simulink model "gm_CSC"  (R2016a)
settings: Solver=FixedStepDiscrete  SolverMode=SingleTasking  StartTime=0.0  StopTime=image_sample_time  RelTol=1e-3
PreLoadFcn:
  | R=105;
  | C=160;
  | Ts = 1/10;
  | image_sample_time = R*C/10;
undefined symbols (not defined in the file or in its folder): gray
libraries: hdlsllib x11, dspsigattribs x2, simulink x2, visionsources x1
Description:
  | Sobel Edge Detection Using the MATLAB(R) Function Block
  | This example shows how to use HDL Coder(TM) to check,
  | generate, and verify HDL code for a Sobel Edge Detection
  | block built using the MATLAB Function block.
settings Model: FPTRunName=Active  Creator=abehbood  LastModifiedBy=KAU-Sprinter
settings DataIOCC: LimitDataPoints=on  SaveFormat=Array  SignalLogging=off
settings OptimizationCC: BlockReduction=off  ConditionallyExecuteInputs=off  DefaultParameterBehavior=Inlined  ExpressionDepthLimit=2147483647  InitFltsAndDblsToZero=on  EfficientMapNaN2IntZero=off
settings DebuggingCC: AlgebraicLoopMsg=error  SaveWithParameterizedLinksMsg=none  UnderspecifiedInitializationDetection=Classic  MergeDetectMultiDrivingBlocksExec=none  SignalResolutionControl=TryResolveAllWithWarning  InheritedTsInSrcMsg=none  MultiTaskDSMMsg=warning  MultiTaskCondExecSysMsg=none  SingleTaskRateTransMsg=error  IntegerOverflowMsg=none  ParameterPrecisionLossMsg=none  FcnCallInpInsideContextMsg=UseLocalSettings  StateNameClashWarn=warning  StrictBusMsg=ErrorOnBusTreatedAsVector  IntegerSaturationMsg=none
settings HardwareCC: ProdBitPerPointer=32  ProdLargestAtomicFloat=None  ProdIntDivRoundTo=Undefined  ProdEndianess=Unspecified  ProdWordSize=32  ProdHWDeviceType=ASIC/FPGA  TargetHWDeviceType=32-bit Generic  ProdEqTarget=off
settings ModelReferenceCC: PropagateSignalLabelsOutOfModel=off
settings GRTTargetCC: TargetFcnLib=ansi_tfl_tmw.mat  CombineOutputUpdateFcns=off  GRTInterface=on
settings ConfigComp: CovModelRefEnable=Off

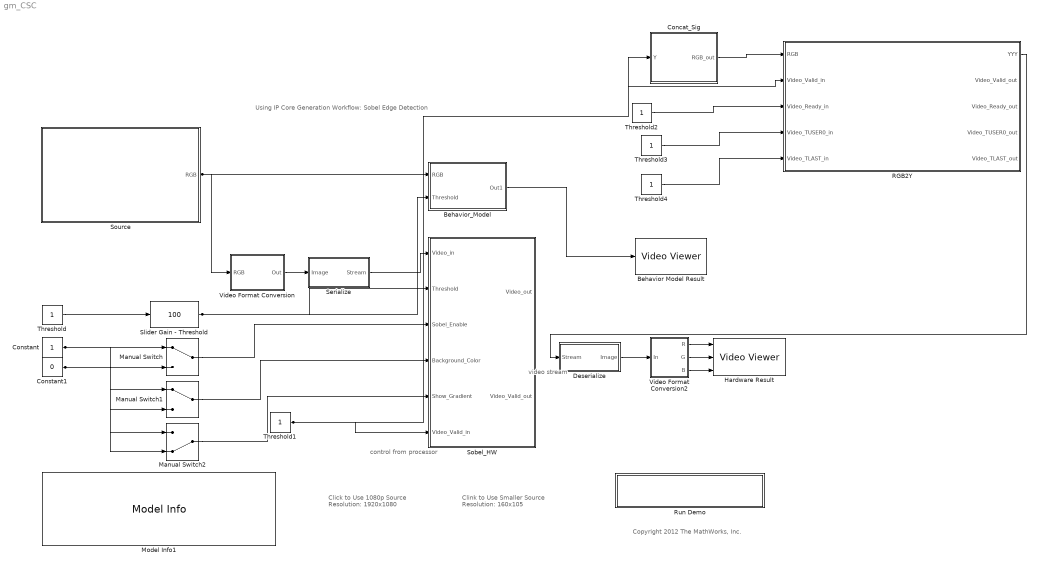
== system gm_CSC ==
  note: control from
      | processor
  note: video
      | stream
  note: Using IP Core Generation Workflow: Sobel Edge Detection
  note: Copyright 2012 The MathWorks, Inc.
  note: Clink to Use Smaller Source
      |
      | Resolution: 160x105
  note: Click to Use 1080p Source
      |
      | Resolution: 1920x1080
  Behavior Model Result : VideoViewer  colormapValue=gray(256)  FigPos=[941 500.4 363.2 159.2]
  Behavior_Model : Subsystem
  Concat_Sig : MATLAB Function  TreatAsAtomicUnit=on
  Constant : Constant  OutDataTypeStr=boolean  SampleTime=Ts
  Constant1 : Constant  Value=0  OutDataTypeStr=boolean  SampleTime=Ts
  Deserialize : Subsystem
  Hardware Result : VideoViewer  imagePorts=separate color signals  colormapValue=gray(256)  FigPos=[1151.4 744.4 360.8 160]
  Manual Switch : ManualSwitch
  Manual Switch1 : ManualSwitch
  Manual Switch2 : ManualSwitch  CurrentSetting=0
  Model Info1 : simulink/Model-Wide Utilities/Model Info  Frame=on  DisplayStringWithTags=|  HorizontalTextAlignment=Left  LeftAlignmentValue=0.02  SourceBlockDiagram=gm_CSC  TagMaxNumber=20
      | This example shows how to use HDL Coder to
      | generate a custom IP core which perform Sobel
      | edge detection processing on streaming video.
      | 
      | In MATLAB, type the following:
      |   hdladvisor('hdlcoder_sobel_video/Sobel_HW')
  RGB2Y : Subsystem  TreatAsAtomicUnit=on
  Run Demo : Subsystem
      settings: OpenFcn=hdladvisor([bdroot, '/Sobel_HW'])
      mask Display: disp('Launch HDL Workflow Advisor')
  Serialize : Subsystem
  Slider Gain - Threshold : simulink/Math Operations/Slider Gain  low=0  gain=100  high=255
  Sobel_HW : Subsystem  TreatAsAtomicUnit=on
  Source : Subsystem
      mask Display: image(imread('hdlcoder_sobel_160_105.jpg'))
  Threshold : Constant  OutDataTypeStr=uint8  SampleTime=Ts
  Threshold{1..4} (4 alike) : Constant  OutDataTypeStr=boolean  SampleTime=Ts
  Video Format Conversion : Subsystem
  Video Format Conversion2 : Subsystem
  wires:
  Threshold4/1 -> RGB2Y/5(Video_TLAST_in)
  Threshold3/1 -> RGB2Y/4(Video_TUSER0_in)
  Threshold2/1 -> RGB2Y/3(Video_Ready_in)
  Concat_Sig/1(RGB_out) -> RGB2Y/1(RGB)
  RGB2Y/1(YYY) -> Deserialize/1(Stream)
  Threshold1/1 -> RGB2Y/2(Video_Valid_in), Sobel_HW/6(Video_Valid_in), Concat_Sig/1(Y)
  Manual Switch2/1 -> Sobel_HW/5(Show_Gradient)
  Manual Switch1/1 -> Sobel_HW/4(Background_Color)
  Manual Switch/1 -> Sobel_HW/3(Sobel_Enable)
  Constant1/1 -> Manual Switch/2, Manual Switch1/2, Manual Switch2/2
  Constant/1 -> Manual Switch/1, Manual Switch1/1, Manual Switch2/1
  Video Format Conversion2/1(R) -> Hardware Result/1
  Video Format Conversion2/2(G) -> Hardware Result/2
  Video Format Conversion2/3(B) -> Hardware Result/3
  Source/1(RGB) -> Video Format Conversion/1(RGB), Behavior_Model/1(RGB)
  Slider Gain - Threshold/1 -> Sobel_HW/2(Threshold), Behavior_Model/2(Threshold)
  Deserialize/1(Image) -> Video Format Conversion2/1(In)
  Video Format Conversion/1(Out) -> Serialize/1(Image)
  Behavior_Model/1(Out1) -> Behavior Model Result/1
  Serialize/1(Stream) -> Sobel_HW/1(Video_in)
  Threshold/1 -> Slider Gain - Threshold/1

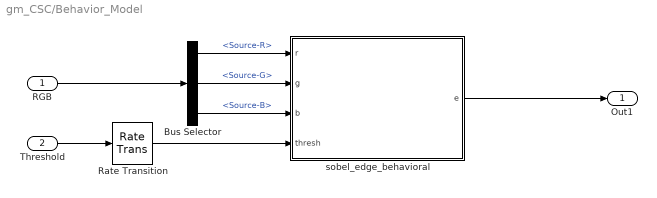
== system gm_CSC/Behavior_Model ==
  RGB : Inport
  Threshold : Inport  Port=2
  Bus Selector : BusSelector  OutputSignals=Source-R,Source-G,Source-B
  Rate Transition : RateTransition
  sobel_edge_behavioral : MATLAB Function  TreatAsAtomicUnit=on
  Out1 : Outport
  wires:
  Rate Transition/1 -> sobel_edge_behavioral/4(thresh)
  Threshold/1 -> Rate Transition/1
  RGB/1 -> Bus Selector/1
  Bus Selector/2 -> sobel_edge_behavioral/2(g)  "<Source-G>"
  Bus Selector/1 -> sobel_edge_behavioral/1(r)  "<Source-R>"
  Bus Selector/3 -> sobel_edge_behavioral/3(b)  "<Source-B>"
  sobel_edge_behavioral/1(e) -> Out1/1

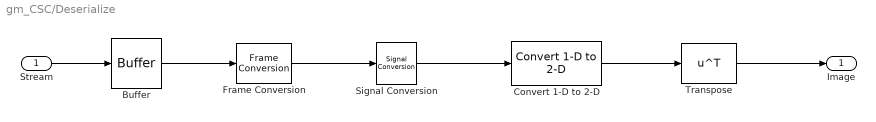
== system gm_CSC/Deserialize ==
  Stream : Inport
  Buffer : Buffer  N=R*C  TreatMby1Signals=One channel
  Convert 1-D to 2-D : dspsigattribs/Convert 1-D to 2-D  M=C  N=R  frameBasedOut=off
  Frame Conversion : FrameConversion  InheritSamplingMode=off  OutFrame=Sample-based
  Signal Conversion : SignalConversion  ConversionOutput=Contiguous copy  OverrideOpt=off
  Transpose : Math  Operator=transpose  SaturateOnIntegerOverflow=on
  Image : Outport
  wires:
  Transpose/1 -> Image/1
  Stream/1 -> Buffer/1
  Convert 1-D to 2-D/1 -> Transpose/1
  Signal Conversion/1 -> Convert 1-D to 2-D/1
  Buffer/1 -> Frame Conversion/1
  Frame Conversion/1 -> Signal Conversion/1

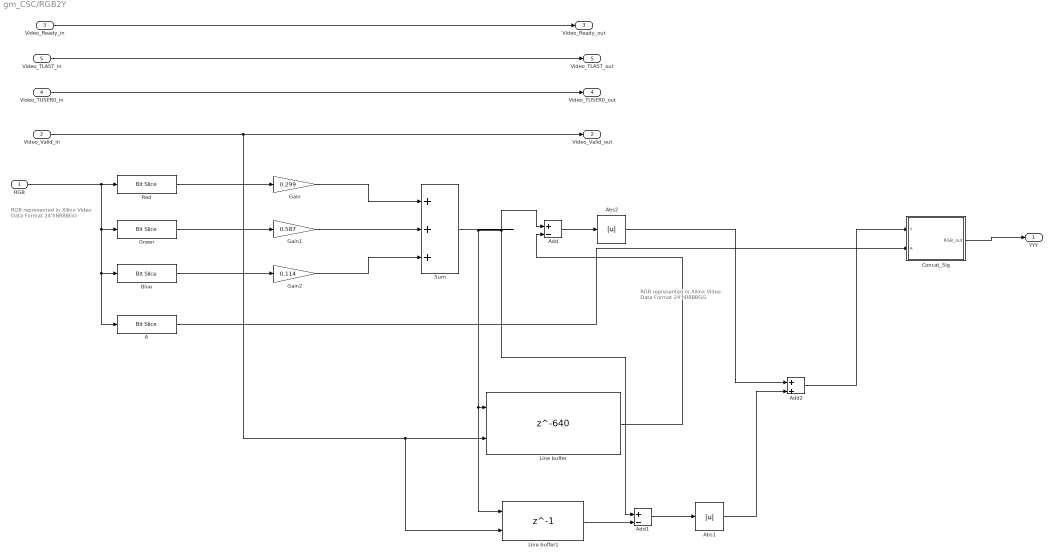
== system gm_CSC/RGB2Y ==
  note: RGB represented in
      | Xilinx Video Data Format
      | 24'hRRBBGG
  note: RGB represented in
      | Xilinx Video Data Format
      | 24'hRRBBGG
  RGB : Inport
  Video_Valid_in : Inport  Port=2
  Video_Ready_in : Inport  Port=3
  Video_TUSER0_in : Inport  Port=4
  Video_TLAST_in : Inport  Port=5
  A : hdlsllib/HDL Operations/Bit Slice  lidx=31  ridx=24
  Abs1 : Abs
  Abs2 : Abs
  Add : Sum  Inputs=+|-  OutDataTypeStr=fixdt(1,12,0)
  Add1 : Sum  Inputs=+|-  OutDataTypeStr=fixdt(1,12,0)
  Add2 : Sum  Inputs=+|+  OutDataTypeStr=fixdt(1,12,0)
  Blue : hdlsllib/HDL Operations/Bit Slice  lidx=15  ridx=8
  Concat_Sig : MATLAB Function  TreatAsAtomicUnit=on
  Gain : Gain  Gain=0.299  OutDataTypeStr=Inherit: Same as input
  Gain1 : Gain  Gain=0.587  OutDataTypeStr=Inherit: Same as input
  Gain2 : Gain  Gain=0.114  OutDataTypeStr=Inherit: Same as input
  Green : hdlsllib/HDL Operations/Bit Slice  lidx=7  ridx=0
  Line buffer : Delay  DelayLength=640  InitialCondition=0  ShowEnablePort=on
      settings: InputPortMap=u0,e6
  Line buffer1 : Delay  DelayLength=1  InitialCondition=0  ShowEnablePort=on
      settings: InputPortMap=u0,e6
  Red : hdlsllib/HDL Operations/Bit Slice  lidx=23  ridx=16
  Sum : Sum  Inputs=+++  OutDataTypeStr=fixdt(1, 9, 0)
  YYY : Outport
  Video_Valid_out : Outport  Port=2
  Video_Ready_out : Outport  Port=3
  Video_TUSER0_out : Outport  Port=4
  Video_TLAST_out : Outport  Port=5
  wires:
  Add2/1 -> Concat_Sig/1(Y)
  Abs2/1 -> Add2/1
  Abs1/1 -> Add2/2
  Add1/1 -> Abs1/1
  Line buffer1/1 -> Add1/2
  Line buffer/1 -> Add/2
  Add/1 -> Abs2/1
  Video_TLAST_in/1 -> Video_TLAST_out/1
  Video_TUSER0_in/1 -> Video_TUSER0_out/1
  Video_Ready_in/1 -> Video_Ready_out/1
  Sum/1 -> Line buffer/1, Line buffer1/1, Add/1, Add1/1
  Video_Valid_in/1 -> Video_Valid_out/1, Line buffer/2, Line buffer1/2
  A/1 -> Concat_Sig/2(A)
  Concat_Sig/1(RGB_out) -> YYY/1
  Blue/1 -> Gain2/1
  Green/1 -> Gain1/1
  Red/1 -> Gain/1
  Gain2/1 -> Sum/3
  Gain1/1 -> Sum/2
  Gain/1 -> Sum/1
  RGB/1 -> Green/1, Blue/1, A/1, Red/1

== system gm_CSC/Run Demo ==

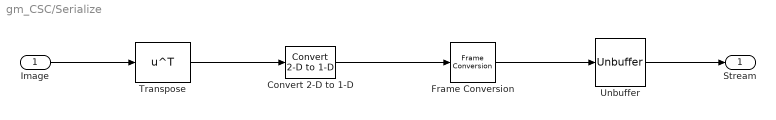
== system gm_CSC/Serialize ==
  Image : Inport
  Convert 2-D to 1-D : dspsigattribs/Convert 2-D to 1-D
  Frame Conversion : FrameConversion  InheritSamplingMode=off
  Transpose : Math  Operator=transpose  SaturateOnIntegerOverflow=on
  Unbuffer : Unbuffer  SampleBasedProcessing=Same as frame based
  Stream : Outport
  wires:
  Unbuffer/1 -> Stream/1
  Frame Conversion/1 -> Unbuffer/1
  Transpose/1 -> Convert 2-D to 1-D/1
  Image/1 -> Transpose/1
  Convert 2-D to 1-D/1 -> Frame Conversion/1

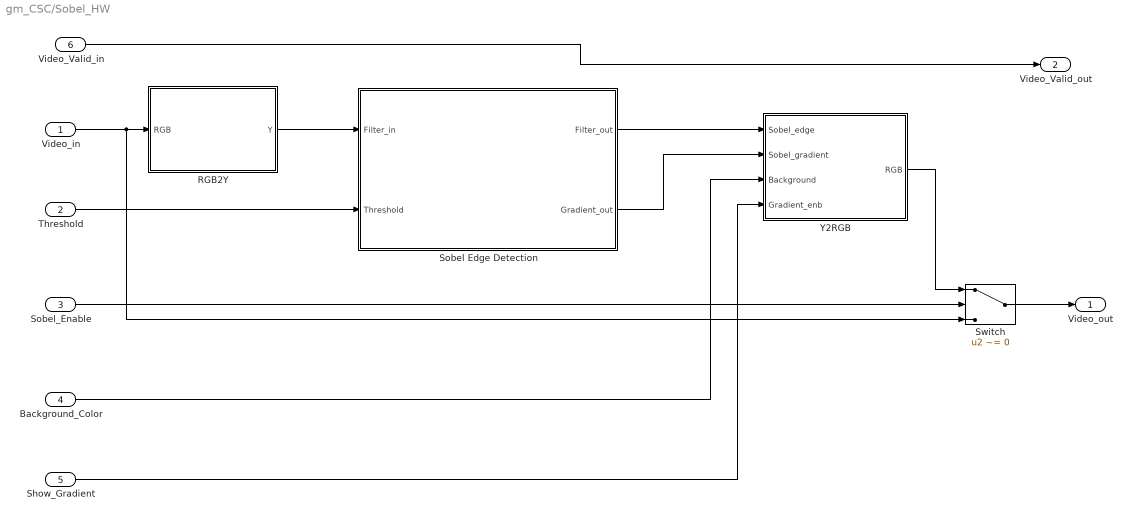
== system gm_CSC/Sobel_HW ==
  Video_in : Inport
  Threshold : Inport  Port=2
  Sobel_Enable : Inport  Port=3
  Background_Color : Inport  Port=4
  Show_Gradient : Inport  Port=5
  Video_Valid_in : Inport  Port=6
  RGB2Y : Subsystem
  Sobel Edge Detection : Subsystem
  Switch : Switch  Criteria=u2 ~= 0
  Y2RGB : Subsystem
  Video_out : Outport
  Video_Valid_out : Outport  Port=2
  wires:
  Video_Valid_in/1 -> Video_Valid_out/1
  Show_Gradient/1 -> Y2RGB/4(Gradient_enb)
  Sobel Edge Detection/2(Gradient_out) -> Y2RGB/2(Sobel_gradient)
  RGB2Y/1(Y) -> Sobel Edge Detection/1("Filter_in ")
  Y2RGB/1(RGB) -> Switch/1
  Background_Color/1 -> Y2RGB/3(Background)
  Sobel Edge Detection/1(Filter_out) -> Y2RGB/1(Sobel_edge)
  Sobel_Enable/1 -> Switch/2
  Switch/1 -> Video_out/1
  Video_in/1 -> RGB2Y/1(RGB), Switch/3
  Threshold/1 -> Sobel Edge Detection/2(Threshold)

== system gm_CSC/Source ==
  Bus Creator : BusCreator  Inputs=3
  Image From File : visionsources/Image From File  Tag=vipblks_nd  FileName=hdlcoder_sobel_160_105.jpg  imagePorts=Separate color signals  Ts=image_sample_time  ImageDataType=uint8  Signed=on  WordLength=16  sdImageDataType=uint(8)  FractionLengthMode=User-defined  FractionLength=15  OutPortLabels=R|G|B
  RGB : Outport
  wires:
  Bus Creator/1 -> RGB/1
  Image From File/1 -> Bus Creator/1  "Source-R"
  Image From File/3 -> Bus Creator/3  "Source-B"
  Image From File/2 -> Bus Creator/2  "Source-G"

== system gm_CSC/Video Format Conversion ==
  note: RGB represented in
      | Xilinx Video Data Format
      | 32'hFFRRBBGG
  RGB : Inport
  Bit Concat : hdlsllib/HDL Operations/Bit Concat  numInputs=4
  Bus Selector : BusSelector  OutputSignals=Source-R,Source-G,Source-B
  White : Constant  Value=255  OutDataTypeStr=uint8  SampleTime=image_sample_time
  Out : Outport
  wires:
  RGB/1 -> Bus Selector/1
  Bus Selector/2 -> Bit Concat/4  "<Source-G>"
  White/1 -> Bit Concat/1
  Bit Concat/1 -> Out/1
  Bus Selector/3 -> Bit Concat/3  "<Source-B>"
  Bus Selector/1 -> Bit Concat/2  "<Source-R>"

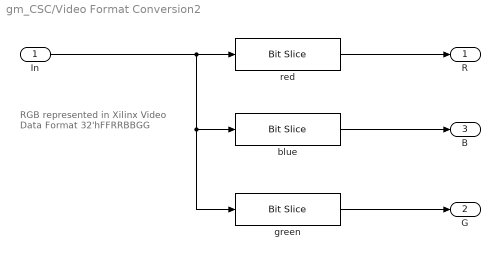
== system gm_CSC/Video Format Conversion2 ==
  note: RGB represented in
      | Xilinx Video Data Format
      | 32'hFFRRBBGG
  In : Inport
  blue : hdlsllib/HDL Operations/Bit Slice  lidx=15  ridx=8
  green : hdlsllib/HDL Operations/Bit Slice  lidx=7  ridx=0
  red : hdlsllib/HDL Operations/Bit Slice  lidx=23  ridx=16
  R : Outport
  G : Outport  Port=2
  B : Outport  Port=3
  wires:
  blue/1 -> B/1
  green/1 -> G/1
  red/1 -> R/1
  In/1 -> red/1, blue/1, green/1

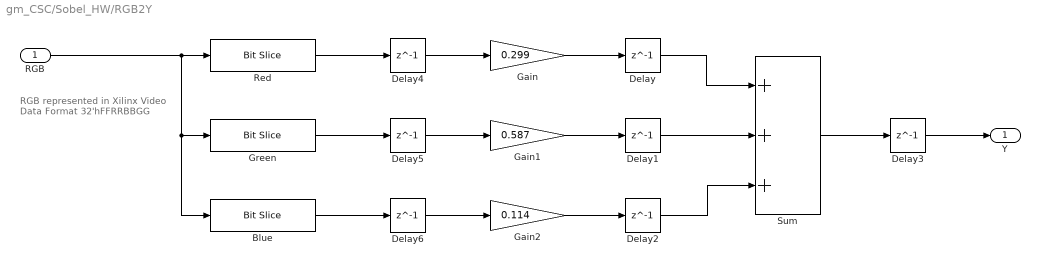
== system gm_CSC/Sobel_HW/RGB2Y ==
  note: RGB represented in
      | Xilinx Video Data Format
      | 32'hFFRRBBGG
  RGB : Inport
  Blue : hdlsllib/HDL Operations/Bit Slice  lidx=15  ridx=8
  Delay{,1..6} (7 alike) : Delay  DelayLength=1  InitialCondition=0
  Gain : Gain  Gain=0.299  OutDataTypeStr=Inherit: Same as input
  Gain1 : Gain  Gain=0.587  OutDataTypeStr=Inherit: Same as input
  Gain2 : Gain  Gain=0.114  OutDataTypeStr=Inherit: Same as input
  Green : hdlsllib/HDL Operations/Bit Slice  lidx=7  ridx=0
  Red : hdlsllib/HDL Operations/Bit Slice  lidx=23  ridx=16
  Sum : Sum  Inputs=+++  OutDataTypeStr=fixdt(1, 9, 0)
  Y : Outport
  wires:
  Delay6/1 -> Gain2/1
  Delay5/1 -> Gain1/1
  Delay4/1 -> Gain/1
  Delay2/1 -> Sum/3
  Delay1/1 -> Sum/2
  Delay/1 -> Sum/1
  Gain1/1 -> Delay1/1
  Gain/1 -> Delay/1
  Sum/1 -> Delay3/1
  Gain2/1 -> Delay2/1
  RGB/1 -> Green/1, Blue/1, Red/1
  Red/1 -> Delay4/1
  Green/1 -> Delay5/1
  Blue/1 -> Delay6/1
  Delay3/1 -> Y/1

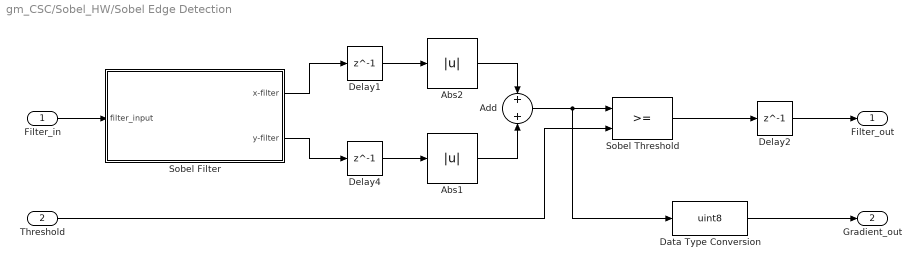
== system gm_CSC/Sobel_HW/Sobel Edge Detection ==
  "Filter_in " : Inport
  Threshold : Inport  Port=2
  Abs1 : Abs
  Abs2 : Abs
  Add : Sum  Inputs=+|+  OutDataTypeStr=fixdt(1,12,0)
  Data Type Conversion : DataTypeConversion  OutDataTypeStr=uint8  SaturateOnIntegerOverflow=on
  Delay1 : Delay  DelayLength=1  InitialCondition=0
  Delay2 : Delay  DelayLength=1  InitialCondition=0
  Delay4 : Delay  DelayLength=1  InitialCondition=0
  Sobel Filter : Subsystem
  Sobel Threshold : RelationalOperator  OutDataTypeStr=boolean
  Filter_out : Outport
  Gradient_out : Outport  Port=2
  wires:
  Data Type Conversion/1 -> Gradient_out/1
  Threshold/1 -> Sobel Threshold/2
  Delay2/1 -> Filter_out/1
  "Filter_in "/1 -> Sobel Filter/1(filter_input)
  Delay4/1 -> Abs1/1
  Sobel Filter/2(y-filter) -> Delay4/1
  Delay1/1 -> Abs2/1
  Sobel Filter/1(x-filter) -> Delay1/1
  Sobel Threshold/1 -> Delay2/1
  Add/1 -> Data Type Conversion/1, Sobel Threshold/1
  Abs2/1 -> Add/1
  Abs1/1 -> Add/2

== system gm_CSC/Sobel_HW/Y2RGB ==
  note: RGB represented in
      | Xilinx Video Data Format
      | 32'hFFRRBBGG
  Sobel_edge : Inport
  Sobel_gradient : Inport  Port=2
  Background : Inport  Port=3
  Gradient_enb : Inport  Port=4
  BW2RGB : MATLAB Function  TreatAsAtomicUnit=on
  RGB : Outport
  wires:
  Gradient_enb/1 -> BW2RGB/4(gradient_enb)
  Sobel_gradient/1 -> BW2RGB/2(sobel_gradient)
  Background/1 -> BW2RGB/3(background_color)
  BW2RGB/1(RGB_out) -> RGB/1
  Sobel_edge/1 -> BW2RGB/1(sobel_edge)

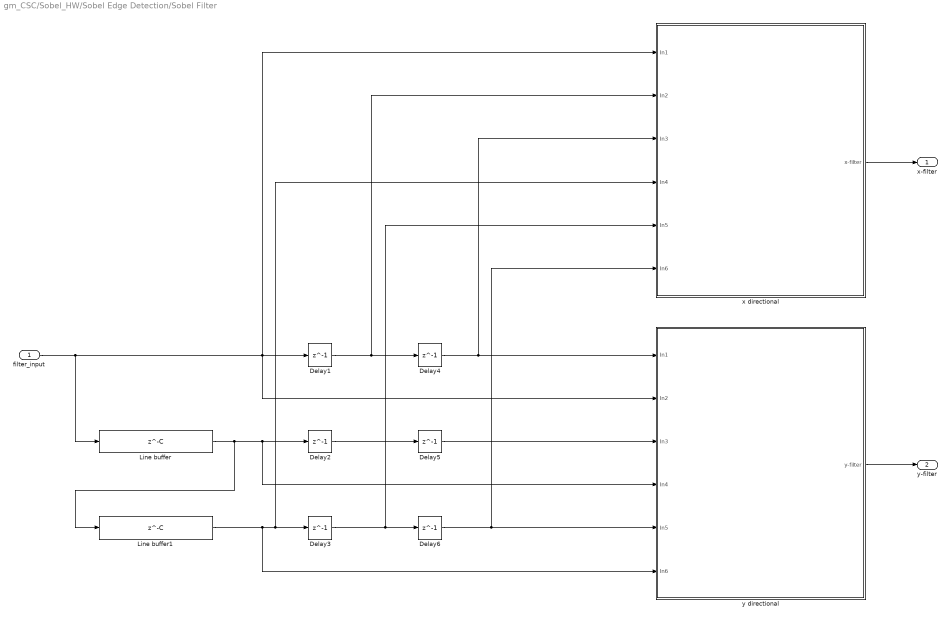
== system gm_CSC/Sobel_HW/Sobel Edge Detection/Sobel Filter ==
  filter_input : Inport
  Delay{1..6} (6 alike) : Delay  DelayLength=1  InitialCondition=0
  Line buffer : Delay  DelayLength=C  InitialCondition=0
  Line buffer1 : Delay  DelayLength=C  InitialCondition=0
  x directional : Subsystem
  y directional : Subsystem
  x-filter : Outport
  y-filter : Outport  Port=2
  wires:
  Delay2/1 -> Delay5/1
  y directional/1(y-filter) -> y-filter/1
  x directional/1(x-filter) -> x-filter/1
  Line buffer1/1 -> y directional/6(In6), x directional/4(In4), Delay3/1
  Line buffer/1 -> y directional/4(In4), Delay2/1, Line buffer1/1
  Delay6/1 -> x directional/6(In6), y directional/5(In5)
  Delay5/1 -> y directional/3(In3)
  Delay3/1 -> x directional/5(In5), Delay6/1
  Delay1/1 -> x directional/2(In2), Delay4/1
  filter_input/1 -> y directional/2(In2), x directional/1(In1), Delay1/1, Line buffer/1
  Delay4/1 -> x directional/3(In3), y directional/1(In1)

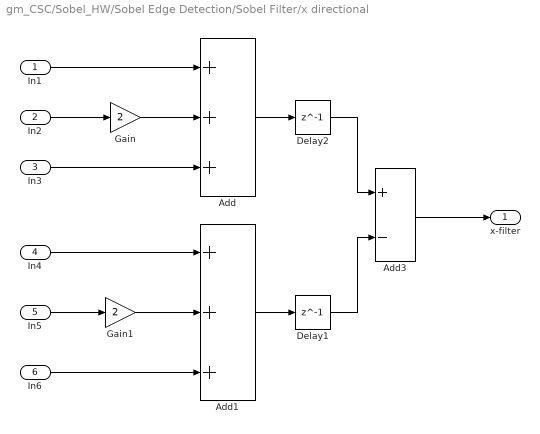
== system gm_CSC/Sobel_HW/Sobel Edge Detection/Sobel Filter/x directional ==
  In1 : Inport
  In2 : Inport  Port=2
  In3 : Inport  Port=3
  In4 : Inport  Port=4
  In5 : Inport  Port=5
  In6 : Inport  Port=6
  Add : Sum  Inputs=+++  OutDataTypeStr=fixdt(1,11,0)
  Add1 : Sum  Inputs=+++  OutDataTypeStr=fixdt(1,11,0)
  Add3 : Sum  Inputs=+-
  Delay1 : Delay  DelayLength=1  InitialCondition=0
  Delay2 : Delay  DelayLength=1  InitialCondition=0
  Gain : Gain  Gain=2  OutDataTypeStr=fixdt(1,10,0)
  Gain1 : Gain  Gain=2  ParamDataTypeStr=sfix(16)  OutDataTypeStr=fixdt(1,10,0)
  x-filter : Outport
  wires:
  Delay1/1 -> Add3/2
  Add1/1 -> Delay1/1
  Delay2/1 -> Add3/1
  Add/1 -> Delay2/1
  Gain1/1 -> Add1/2
  In6/1 -> Add1/3
  In5/1 -> Gain1/1
  In4/1 -> Add1/1
  In3/1 -> Add/3
  Gain/1 -> Add/2
  Add3/1 -> x-filter/1
  In2/1 -> Gain/1
  In1/1 -> Add/1

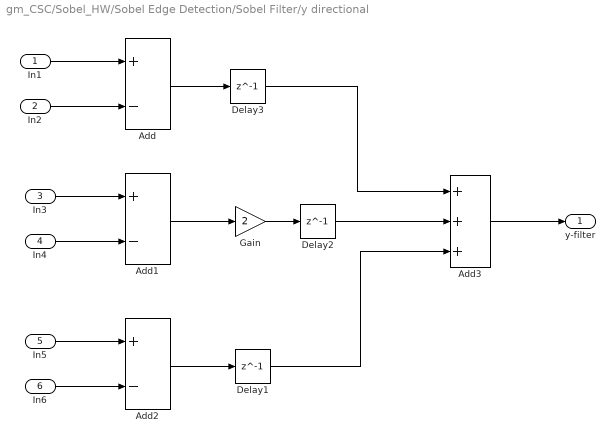
== system gm_CSC/Sobel_HW/Sobel Edge Detection/Sobel Filter/y directional ==
  In1 : Inport
  In2 : Inport  Port=2
  In3 : Inport  Port=3
  In4 : Inport  Port=4
  In5 : Inport  Port=5
  In6 : Inport  Port=6
  Add : Sum  Inputs=+-  OutDataTypeStr=fixdt(1,11,0)
  Add1 : Sum  Inputs=+-  OutDataTypeStr=fixdt(1,11,0)
  Add2 : Sum  Inputs=+-  OutDataTypeStr=fixdt(1,11,0)
  Add3 : Sum  Inputs=+++
  Delay1 : Delay  DelayLength=1  InitialCondition=0
  Delay2 : Delay  DelayLength=1  InitialCondition=0
  Delay3 : Delay  DelayLength=1  InitialCondition=0
  Gain : Gain  Gain=2  OutDataTypeStr=fixdt(1,11,0)
  y-filter : Outport
  wires:
  Delay2/1 -> Add3/2
  Gain/1 -> Delay2/1
  Delay1/1 -> Add3/3
  Add2/1 -> Delay1/1
  Delay3/1 -> Add3/1
  Add/1 -> Delay3/1
  In5/1 -> Add2/1
  In3/1 -> Add1/1
  In1/1 -> Add/1
  In6/1 -> Add2/2
  In4/1 -> Add1/2
  In2/1 -> Add/2
  Add1/1 -> Gain/1
  Add3/1 -> y-filter/1

== matlab function gm_CSC/RGB2Y/Concat_Sig ==
  data: Y input; RGB_out output; A input
function RGB_out = Concat_Sig(Y,A)
% 32'hAARRBBGG

Rd = fi(Y, 0, 8, 0);
Gr = fi(Y, 0, 8, 0);
Bl = fi(Y, 0, 8, 0);
AA = fi(A, 0, 8, 0);
RGB_out = bitconcat(AA,Rd,Gr,Bl);

== matlab function gm_CSC/Behavior_Model/sobel_edge_behavioral ==
  data: r input uint8; g input uint8; b input uint8; e output; thresh input uint8
function e = fcn(r, g, b, thresh)
% SOBEL EDGE DETECTION
%
% Edges characterize boundaries and are therefore a problem of fundamental 
% importance in image processing. Edges in images are areas with strong 
% intensity contrasts. Edge detecting an image significantly 
% reduces the amount of data and filters out useless information, 
% while preserving the important structural properties in an image. 

% The Sobel operator performs a 2-D spatial gradient measurement on an 
% image. Typically it is used to find the approximate absolute gradient 
% magnitude at each point in an input grayscale image. The Sobel edge 
% detector uses a pair of 3x3 convolution masks, one estimating the 
% gradient in the x-direction (columns) and the other estimating the 
% gradient in the y-direction (rows). A convolution mask is usually much 
% smaller than the actual image. As a result, the mask is slid over the 
% image, manipulating a square of pixels at a time. The actual Sobel 
% masks are shown below

u = r * 0.299 + g * 0.587 + b * 0.114;

% Note that 'gy' is simply 'gx' rotated 90deg anti clockwise
gx = [-1,  0,  1; 
      -2,  0,  2; 
      -1,  0,  1];
  
gy = [ 1,  2,  1;  
       0,  0,  0; 
      -1, -2, -1];

a1t = abs(conv2(gx, double(u), 'full'));
a2t = abs(conv2(gy, double(u), 'full'));

a1 = a1t(3:end-2, 3:end-2);
a2 = a2t(3:end-2, 3:end-2);

% The masks are designed to respond maximally to edges 
% running vertically and horizontally relative to the pixel grid, 
% one mask for each of the two perpendicular orientations. 
% The masks can be applied separately to the input image, 
% to produce separate measurements of the gradient component 
% in each orientation (call these Gx and Gy). These can then 
% be combined together to find the absolute magnitude of the 
% gradient at each point and the orientation of that gradient. 
% The gradient magnitude is given by
%  |G| = sqrt((gx * u)^2 + (gy * u)^2)

e = sqrt(a1 .* a1 + a2 .* a2) >= thresh;

== matlab function gm_CSC/Sobel_HW/Y2RGB/BW2RGB ==
  data: sobel_edge input boolean; sobel_gradient input uint8; RGB_out output; background_color input boolean; gradient_enb input boolean
function RGB_out = BW2RGB(sobel_edge, sobel_gradient, background_color, gradient_enb)
% DisplaRGB_out sobel output (black or white) in RGB format.
% RGB is represented in Xilinx Video Data Format Representation
% 32'hFFRRBBGG

black = fi(0, 0, 8, 0);
white = fi(255, 0, 8, 0);
RGB_white = bitconcat(white, white, white, white);
RGB_black = bitconcat(white, black, black, black);

% RGB format must start with FF
if gradient_enb
    intensity = fi(sobel_gradient, 0, 8, 0);
    RGB_out = bitconcat(white, intensity, intensity, intensity);
else
    if background_color
        % background_color = 1, background is black
        if sobel_edge
            RGB_out = RGB_white;
        else
            RGB_out = RGB_black;
        end
    else
        % background_color = 0, background is white
        if sobel_edge
            RGB_out = RGB_black;
        else
            RGB_out = RGB_white;
        end
    end
end

== matlab function gm_CSC/Concat_Sig ==
  data: Y input boolean; RGB_out output
function RGB_out = Concat_Sig_Out(Y)
% 32'hAARRBBGG

Aa = fi(0, 0, 8, 0);
Rd = fi(0, 0, 8, 0);
Gr = fi(0, 0, 8, 0);
Bl = fi(0, 0, 8, 0);

RGB_out = bitconcat(Aa,Rd,Gr,Bl);
